simulink model "ofb"  (Simulink 7.8)
settings: Solver=ode45  StartTime=0.0  StopTime=1e-1  RelTol=1e-3
values from neighbouring files (symbols this model uses):
  corrmagnetgain = param.corrmagnetgain    [simfofb.m]
  fofbctrl = param.fofbctrl    [simfofb.m]
  ncorrfofb = size(fofbctrl.sys.d, 1)    [simfofb.m]    (also in simfofb_lnls1.m = size(param.fofbctrl.sys.d, 1); simfofb_sirius.m = size(param.fofbctrl.sys.d, 1))
  ncorrsofb = size(sofbctrl.sys.d, 1)    [simfofb.m]    (also in simfofb_lnls1.m = 1; simfofb_sirius.m = 1)
  sofbctrl = param.sofbctrl    [simfofb.m]
undefined symbols (not defined in the file or in its folder): fracnetdelay
libraries: cstblocks x5
settings Model: Creator=daniel.tavares  LastModifiedBy=danielot
settings DataIOCC: ExternalInput=[simvectors.t simvectors.reference_orbit simvectors.orbit_distortion simvectors.sofb_setpoints simvectors.fofb_setpoints simvectors.bpm_noise simvectors.corrsofb_current_noise simvectors.corrsofb_power_noise]  LimitDataPoints=off  LoadExternalInput=on  SaveFormat=StructureWithTime  SignalLogging=off  DSMLogging=off
settings DebuggingCC: AlgebraicLoopMsg=none  ArtificialAlgebraicLoopMsg=none

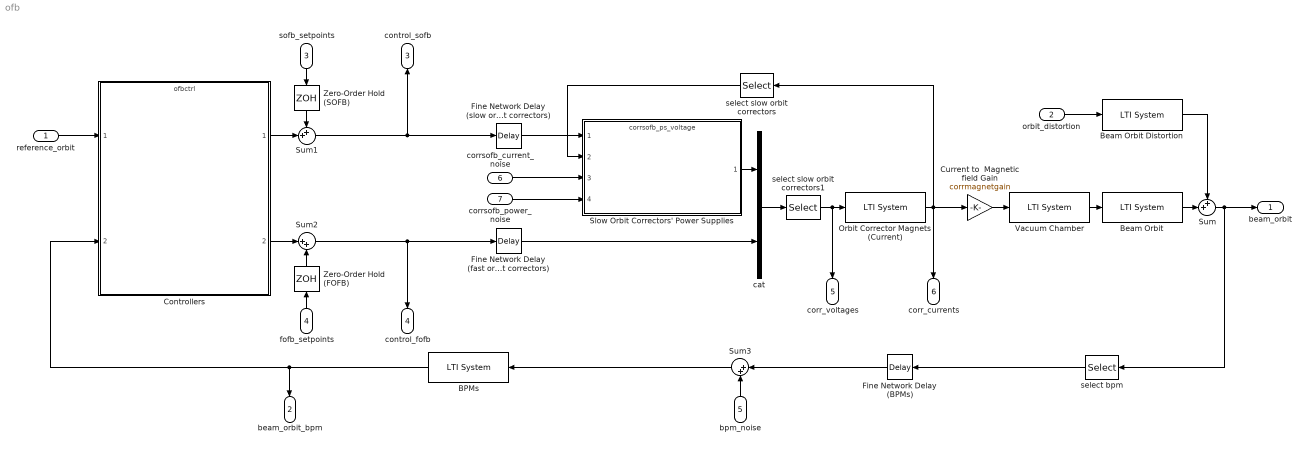
== system ofb ==
  reference_orbit : Inport  PortDimensions=nbpm
  orbit_distortion : Inport  Port=2  PortDimensions=ndist
  sofb_setpoints : Inport  Port=3  PortDimensions=ncorrsofb
  fofb_setpoints : Inport  Port=4  PortDimensions=ncorrfofb
  bpm_noise : Inport  Port=5  PortDimensions=nbpm
  corrsofb_current_noise : Inport  Port=6  PortDimensions=ncorrsofb
  corrsofb_power_noise : Inport  Port=7  PortDimensions=ncorrsofb
  BPMs : cstblocks/LTI System  sys=bpm.sys  IC=[]
  Beam Orbit : cstblocks/LTI System  sys=beam.sys  IC=[]
  Beam Orbit Distortion : cstblocks/LTI System  sys=distbeam.sys  IC=[]
  Controllers : ModelReference  ModelNameDialog=ofbctrl  SimulationMode=Accelerator  ModelReferenceVersion=1.203  CopyOfModelName=ofbctrl  DefaultDataLogging=on
  Current to  Magnetic field Gain : Gain  Gain=corrmagnetgain
  Fine Network Delay (BPMs) : TransportDelay  DelayTime=fracnetdelay.bpm  TransDelayFeedthrough=on
  Fine Network Delay (fast orbit correctors) : TransportDelay  DelayTime=fracnetdelay.corrfofb  TransDelayFeedthrough=on
  Fine Network Delay (slow orbit correctors) : TransportDelay  DelayTime=fracnetdelay.corrsofb  TransDelayFeedthrough=on
  Orbit Corrector Magnets (Current) : cstblocks/LTI System  sys=corrmagnet.sys  IC=[]
  Slow Orbit Correctors' Power Supplies : ModelReference  ModelNameDialog=corrsofb_ps_voltage.mdl  SimulationMode=Accelerator  ModelReferenceVersion=1.18  CopyOfModelName=corrsofb_ps_voltage.mdl  DefaultDataLogging=on
  Sum : Sum  Inputs=++|
  Sum1 : Sum  Inputs=++|
  Sum2 : Sum  Inputs=|++
  Sum3 : Sum  Inputs=|++
  Vacuum Chamber : cstblocks/LTI System  sys=vacchamb.sys  IC=[]
  Zero-Order Hold (FOFB) : ZeroOrderHold  SampleTime=fofbctrl.sys.Ts
  Zero-Order Hold (SOFB) : ZeroOrderHold  SampleTime=sofbctrl.sys.Ts
  cat : Concatenate  Mode=Vector
  select bpm : Selector  InputPortWidth=norbit  IndexOptions=Index vector (dialog)  Indices=bpmselect  OutputSizes=1
  select slow orbit correctors : Selector  InputPortWidth=ncorr  IndexOptions=Index vector (dialog)  Indices=corrsofbselect  OutputSizes=1
  select slow orbit correctors1 : Selector  InputPortWidth=ncorrsofb+ncorrfofb  IndexOptions=Index vector (dialog)  Indices=corrordering  OutputSizes=1
  beam_orbit : Outport
  beam_orbit_bpm : Outport  Port=2
  control_sofb : Outport  Port=3
  control_fofb : Outport  Port=4
  corr_voltages : Outport  Port=5
  corr_currents : Outport  Port=6
  wires:
  Beam Orbit/1 -> Sum/2
  orbit_distortion/1 -> Beam Orbit Distortion/1
  bpm_noise/1 -> Sum3/2
  Vacuum Chamber/1 -> Beam Orbit/1
  Beam Orbit Distortion/1 -> Sum/1
  Sum/1 -> beam_orbit/1, select bpm/1
  Orbit Corrector Magnets (Current)/1 -> select slow orbit correctors/1, Current to  Magnetic field Gain/1, corr_currents/1
  Sum3/1 -> BPMs/1
  Current to  Magnetic field Gain/1 -> Vacuum Chamber/1
  Fine Network Delay (fast orbit correctors)/1 -> cat/2
  reference_orbit/1 -> Controllers/1
  cat/1 -> select slow orbit correctors1/1
  Slow Orbit Correctors' Power Supplies/1 -> cat/1
  corrsofb_power_noise/1 -> Slow Orbit Correctors' Power Supplies/4
  corrsofb_current_noise/1 -> Slow Orbit Correctors' Power Supplies/3
  select slow orbit correctors/1 -> Slow Orbit Correctors' Power Supplies/2
  Fine Network Delay (slow orbit correctors)/1 -> Slow Orbit Correctors' Power Supplies/1
  select slow orbit correctors1/1 -> corr_voltages/1, Orbit Corrector Magnets (Current)/1
  Controllers/1 -> Sum1/2
  Sum1/1 -> Fine Network Delay (slow orbit correctors)/1, control_sofb/1
  sofb_setpoints/1 -> Zero-Order Hold (SOFB)/1
  Controllers/2 -> Sum2/1
  fofb_setpoints/1 -> Zero-Order Hold (FOFB)/1
  Sum2/1 -> Fine Network Delay (fast orbit correctors)/1, control_fofb/1
  Fine Network Delay (BPMs)/1 -> Sum3/1
  BPMs/1 -> Controllers/2, beam_orbit_bpm/1
  Zero-Order Hold (SOFB)/1 -> Sum1/1
  Zero-Order Hold (FOFB)/1 -> Sum2/2
  select bpm/1 -> Fine Network Delay (BPMs)/1
